simulink model "CasaDi_NMPC_MHE_UGV_circle2m"  (R2022a)
settings: Solver=VariableStepAuto  StartTime=0.0  StopTime=60*2  RelTol=1e-3
values from neighbouring files (symbols this model uses):
  L = 0.14    [MHE_RK_CasaDi.m]    (also in NonLinear_MPC_with_Obstacles_CasaDi.m; SimulationParameters.mat)
  Optitrack_meanerr = [0 0 0]    [SimulationParameters.mat]
  Optitrack_Ts = 0.00833333333333    [SimulationParameters.mat]
  Optitrack_var = [2e-05 2e-05 0.00174532925199]    [SimulationParameters.mat]
  Ts = 0.1    [MHE_RK_CasaDi.m]    (also in NonLinear_MPC_with_Obstacles_CasaDi.m; SimulationParameters.mat)
settings Model: Creator=mrnel  LastModifiedBy=root

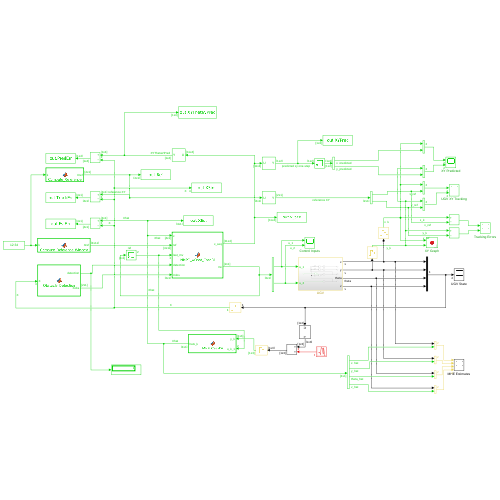
[thumbnail: Simulink's stored preview of the top-level diagram]
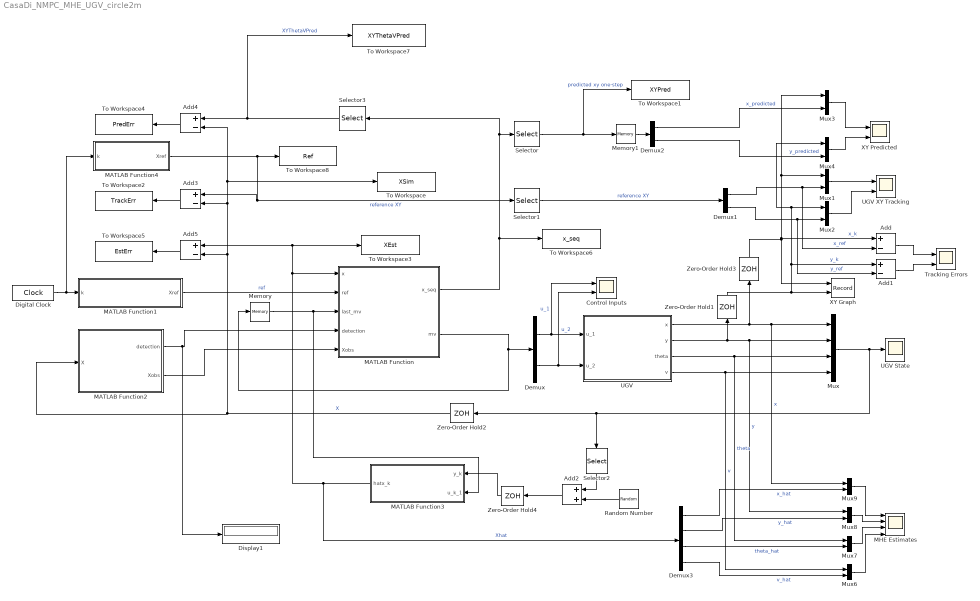
== system CasaDi_NMPC_MHE_UGV_circle2m ==
  Add{,1,3..5} (5 alike) : Sum  Inputs=+-
  Add2 : Sum
  Control Inputs : Scope  NumInputPorts=2
  Demux : Demux  Outputs=2
  Demux1 : Demux  Outputs=2
  Demux2 : Demux  Outputs=2
  Demux3 : Demux
  Digital Clock : DigitalClock  SampleTime=Ts
  Display1 : Display
  MATLAB Function : MATLAB Function  TreatAsAtomicUnit=on  SystemSampleTime=Ts
  MATLAB Function1 : MATLAB Function  TreatAsAtomicUnit=on  SystemSampleTime=Ts
  MATLAB Function2 : MATLAB Function  TreatAsAtomicUnit=on  SystemSampleTime=Ts
  MATLAB Function3 : MATLAB Function  TreatAsAtomicUnit=on  SystemSampleTime=Ts
  MATLAB Function4 : MATLAB Function  TreatAsAtomicUnit=on  SystemSampleTime=Ts
  MHE Estimates : Scope  NumInputPorts=4
  Memory : Memory  InitialCondition=[0;0]  InheritSampleTime=on
  Memory1 : Memory  InitialCondition=[2,0]  InheritSampleTime=on
  Mux : Mux
  Mux{1..4,6..9} (8 alike) : Mux  Inputs=2
  Random Number : RandomNumber  Mean=Optitrack_meanerr  Variance=Optitrack_var.^2  SampleTime=Optitrack_Ts
  Selector : Selector  NumberOfDimensions=2  InputPortWidth=3  IndexOptions=Index vector (dialog),Index vector (dialog)  Indices=2,[1 2]  OutputSizes=1,1
  Selector1 : Selector  NumberOfDimensions=2  InputPortWidth=3  IndexOptions=Index vector (dialog),Index vector (dialog)  Indices=[1 2 ],1  OutputSizes=1,1
  Selector2 : Selector  NumberOfDimensions=2  InputPortWidth=3  IndexOptions=Index vector (dialog),Index vector (dialog)  Indices=1,[1:3]  OutputSizes=1,1
  Selector3 : Selector  NumberOfDimensions=2  InputPortWidth=3  IndexOptions=Index vector (dialog),Select all  Indices=2,[1 2]  OutputSizes=1,1
  To Workspace : ToWorkspace  VariableName=XSim  SaveFormat=Timeseries  SampleTime=Ts
  To Workspace1 : ToWorkspace  VariableName=XYPred  SaveFormat=Timeseries  SampleTime=Ts
  To Workspace2 : ToWorkspace  VariableName=TrackErr  SaveFormat=Timeseries  SampleTime=Ts
  To Workspace3 : ToWorkspace  VariableName=XEst  SaveFormat=Timeseries  SampleTime=Ts
  To Workspace4 : ToWorkspace  VariableName=PredErr  SaveFormat=Timeseries  SampleTime=Ts
  To Workspace5 : ToWorkspace  VariableName=EstErr  SaveFormat=Timeseries  SampleTime=Ts
  To Workspace6 : ToWorkspace  VariableName=x_seq  SaveFormat=Timeseries  SampleTime=-1
  To Workspace7 : ToWorkspace  VariableName=XYThetaVPred  SaveFormat=Timeseries  SampleTime=Ts
  To Workspace8 : ToWorkspace  VariableName=Ref  SaveFormat=Timeseries  SampleTime=Ts
  Tracking Errors : Scope  NumInputPorts=2
  UGV : Subsystem
  UGV State : Scope
  UGV XY Tracking : Scope  NumInputPorts=2
  XY Graph : Record  FileSettingsInternal="{\"entries\":[{\"content\":{\"excelSettings\":{\"content\":{},\"type\":\"Streamout.ExcelSettings\"}},\"type\":\"Streamout.FileSettingStorage\",\"uuid\":\"\"}],\"packageUris\":[\"http:\\/\\/schema.mathworks.com\\/mf0\\/streamout_blocks\\/R2020a\"],\"version\":\"1.0\"}"  Layout=[1 1]  SignalsInternal="{\"entries\":[{\"content\":{\"signals\":[{\"content\":{\"blockPath\":[],\"channel\":[],\"dimensions\":[1,1],\"domain\":\"\",\"lineColor\":\"#a2142f\",\"plots\":[],\"port\":1,\"sid\":[\"\"],\"signalID\":288,\"signalName\":\"x_k\"},\"type\":\"RecordBlkView.Signal\",\"uuid\":\"\"},{\"content\":{\"blockPath\":[],\"channel\":[],\"dimensions\":[1,1],\"domain\":\"\",\"lineColor\":\"#139fff\",\"plots\":[],\"port\":2,\"sid\":[\"\"],\"signalID\":292,\"signalName\":\"y_k\"},\"type\":\"RecordBlkView.Signal\",\"uuid\":\"\"}]},\"type\":\"RecordBlkView.InputSignals\",\"uuid\":\"\"}],\"packageUris\":[\"http:\\/\\/schema.mathworks.com\\/mf0\\/streamout_blocks\\/R2020a\"],\"version\":\"1.0\"}"  VisualizationBindings="{\"xyplotplugin\":{\"info\":[{\"series\":[],\"subplotID\":1}]}}"  CompatibilityTag=XY
  XY Predicted : Scope  NumInputPorts=2
  Zero-Order Hold1 : ZeroOrderHold  SampleTime=Ts
  Zero-Order Hold2 : ZeroOrderHold  SampleTime=Ts
  Zero-Order Hold3 : ZeroOrderHold  SampleTime=Ts
  Zero-Order Hold4 : ZeroOrderHold  SampleTime=0.1
  wires:
  Demux/1 -> UGV/1(u_1), Control Inputs/1  "u_1"
  Demux/2 -> UGV/2("u_2 "), Control Inputs/2  "u_2"
  MATLAB Function/2(mv) -> Demux/1, Memory/1
  Mux/1 -> UGV State/1, Zero-Order Hold2/1, Selector2/1
  Memory/1 -> MATLAB Function3/2(u_k_1), MATLAB Function/3(last_mv)
  UGV/1(x) -> Mux/1, Mux9/1, Zero-Order Hold3/1  "x"
  UGV/2(y) -> Mux/2, Mux8/1, Zero-Order Hold1/1  "y"
  UGV/3(theta) -> Mux/3, Mux7/1  "theta"
  UGV/4(v) -> Mux/4, Mux6/1  "v"
  MATLAB Function/1(x_seq) -> To Workspace6/1, Selector3/1, Selector/1
  Selector/1 -> Memory1/1, To Workspace1/1  "predicted xy one-step"
  Digital Clock/1 -> MATLAB Function4/1(k), MATLAB Function1/1(k)
  Selector1/1 -> Demux1/1  "reference XY"
  Demux2/1 -> Mux3/2  "x_predicted"
  Demux2/2 -> Mux4/2  "y_predicted"
  Mux4/1 -> XY Predicted/2
  Mux3/1 -> XY Predicted/1
  Mux1/1 -> UGV XY Tracking/1
  Mux2/1 -> UGV XY Tracking/2
  Demux1/1 -> Add/2, Mux1/2  "x_ref"
  Demux1/2 -> Mux2/2, Add1/2  "y_ref"
  Zero-Order Hold1/1 -> XY Graph/2, Add1/1, Mux4/1, Mux2/1  "y_k"
  Zero-Order Hold3/1 -> XY Graph/1, Mux3/1, Mux1/1, Add/1  "x_k"
  Add/1 -> Tracking Errors/1
  Add1/1 -> Tracking Errors/2
  MATLAB Function3/1(hatx_k) -> Demux3/1, To Workspace3/1, Add5/1, MATLAB Function/1(x)  "Xhat"
  Add2/1 -> Zero-Order Hold4/1
  Random Number/1 -> Add2/2
  Zero-Order Hold4/1 -> MATLAB Function3/1(y_k)
  Selector2/1 -> Add2/1
  Demux3/1 -> Mux9/2  "x_hat"
  Demux3/2 -> Mux8/2  "y_hat"
  Demux3/3 -> Mux7/2  "theta_hat"
  Demux3/4 -> Mux6/2  "v_hat"
  Mux9/1 -> MHE Estimates/1
  Mux8/1 -> MHE Estimates/2
  Mux7/1 -> MHE Estimates/3
  Mux6/1 -> MHE Estimates/4
  Memory1/1 -> Demux2/1
  Add4/1 -> To Workspace4/1
  Add5/1 -> To Workspace5/1
  Zero-Order Hold2/1 -> Add5/2, Add3/2, To Workspace/1, Add4/2, MATLAB Function2/1(X)  "X"
  Selector3/1 -> To Workspace7/1, Add4/1  "XYThetaVPred"
  MATLAB Function2/1(detection) -> Display1/1, MATLAB Function/4(detection)
  MATLAB Function2/2(Xobs) -> MATLAB Function/5(Xobs)
  MATLAB Function1/1(Xref) -> MATLAB Function/2(ref)  "ref"
  Add3/1 -> To Workspace2/1
  MATLAB Function4/1(Xref) -> To Workspace8/1, Add3/1, Selector1/1  "reference XY"

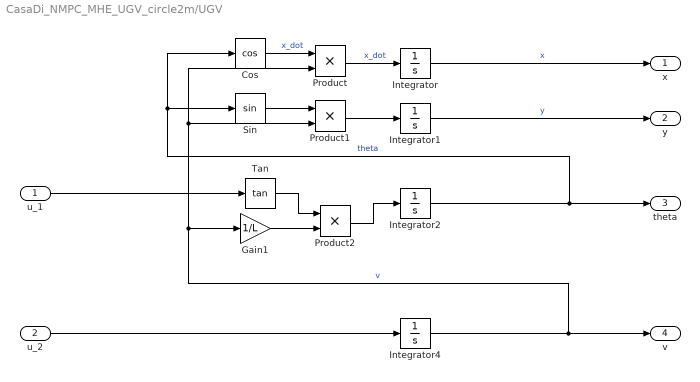
== system CasaDi_NMPC_MHE_UGV_circle2m/UGV ==
  u_1 : Inport
  "u_2 " : Inport  Port=2
  Cos : Trigonometry  Operator=cos
  Gain1 : Gain  Gain=1/L
  Integrator : Integrator  InitialCondition=2
  Integrator1 : Integrator
  Integrator2 : Integrator  InitialCondition=pi/2
  Integrator4 : Integrator  LimitOutput=on  UpperSaturationLimit=1  LowerSaturationLimit=-1
  Product : Product
  Product1 : Product
  Product2 : Product
  Sin : Trigonometry
  Tan : Trigonometry  Operator=tan
  x : Outport
  y : Outport  Port=2
  theta : Outport  Port=3
  v : Outport  Port=4
  wires:
  Product2/1 -> Integrator2/1
  Product1/1 -> Integrator1/1
  Cos/1 -> Product/1  "x_dot"
  Sin/1 -> Product1/1
  Tan/1 -> Product2/1
  Product/1 -> Integrator/1  "x_dot"
  Integrator4/1 -> Product1/2, Product/2, Gain1/1, v/1  "v"
  u_1/1 -> Tan/1
  Integrator1/1 -> y/1  "y"
  "u_2 "/1 -> Integrator4/1
  Integrator/1 -> x/1  "x"
  Integrator2/1 -> Cos/1, Sin/1, theta/1  "theta"
  Gain1/1 -> Product2/2

== matlab function CasaDi_NMPC_MHE_UGV_circle2m/MATLAB Function1 ==
  settings: updateMethod=DISCRETE  sampleTime=Ts
  data: Xref output; k input
function Xref = Compute_Reference_Window(k)
%COMPUTE_REFERENCE_WINDOW This function computes the reference over the prediction
%window, i.e., for instants k, k+1, ..., k+Hp

% Prediction horizon
Hp = 10;

% Time instants over the prediction horizon
time_horizon = k + 0.1 * (0:Hp);

% Intialization of the memory with zeros
Xref = zeros(4,Hp+1);

% Circular trajectory reference for pose and forward velocity. 
w = 2*pi/(60);
Xref = [2*cos(time_horizon*w);
        2*sin(time_horizon*w);
        w*time_horizon+(pi/2);
        2*w*ones(1,Hp+1)];

== matlab function CasaDi_NMPC_MHE_UGV_circle2m/MATLAB Function ==
  data: x input; ref input; last_mv input; x_seq output; mv output; detection input; Xobs input
function [x_seq, mv] = NMPC_wObst_CasaDi(x, ref, last_mv, ...
    detection, Xobs)
%NMPC_WOBST_CASADI This function calls the NMPC function. In particular the
% NMPC formulation includes constraints for obstacle avoidance and the IPOPT
% solver is used to solve the nonlinear optimization problem

% In order to call the 'NonLinear_MPC_with_Obstacles_CasaDi' MATLAB
% Function with the CasaDi library functions calls.
coder.extrinsic("NonLinear_MPC_with_Obstacles_CasaDi");

% Prediction horizon
Hp = 10;

% N. of state variables
n_states = 4;

% N. of control variables
n_controls = 2;

% Initialization of the the memory with zeros of the return values, i.e.,
% * the optimal state sequence over the prediction horizon
x_seq = zeros(Hp+1,n_states);

% * the optimal first control value from the optimal control sequenceover
% the control horizon
mv = zeros(n_controls,1);

% Call of the 'NonLinear_MPC_with_Obstacles_CasaDi' MATLAB function
[x_seq, mv] = NonLinear_MPC_with_Obstacles_CasaDi(x, ref, last_mv, ...
    detection, Xobs);

== matlab function CasaDi_NMPC_MHE_UGV_circle2m/MATLAB Function2 ==
  settings: updateMethod=DISCRETE  sampleTime=Ts
  data: detection output; X input; Xobs output
function [detection, Xobs] = Obstacle_Detection(X)
%OBSTACLE_DETECTION This function implements in some sort the logic of the
% LiDar sensor assumed to be included in the onboard equipment.For
% debugging, a warning is through in case the vehicle enters in the unsafe
% region (i.e., it's too close to the vehicle).

% In order to through a warning if the safety region is not respected
% (i.e., too close to the obstacle)
coder.extrinsic('warning')

% The unknown obstacle is splaced in (x,y) = (-2,0)
Xobs = [-2;0];

% Flag whether an obstacle is detected, 1, or not, 0. By default, no
% obstacle is detected by the LiDar sensor
detection = 0;

% Range of the LiDar sensor.
d_LiDar = 5;%[m]

% Safety distance that the vehicle should keep from the obstacle
d_SAFE = 0.25;%[m]

% If the LiDar onboard detects an obstacle
if norm(X(1:2)-Xobs) < d_LiDar
    % Update the flag 
    detection = 1;
    % If the vehicle enters in the unsafe region ...
    if norm(X(1:2)-Xobs) < d_SAFE
        % ...through a warning...
        warning('too close the obstacle');
        % ...and display the distance from the obstacle (for debugging)
        disp(norm(X(1:2)-Xobs));
    end
end

== matlab function CasaDi_NMPC_MHE_UGV_circle2m/MATLAB Function3 ==
  data: y_k input; hatx_k output; u_k_1 input
function hatx_k = MHE_CasaDi(y_k , u_k_1)
%MHE_CASADI This function calls the MHE function. In particular the IPOPT
% solver is used to solve the nonlinear optimization problem

% In order to call the 'MHE_RK_CasaDi' MATLAB function with the CasaDi 
% library functions calls.
coder.extrinsic("MHE_RK_CasaDi");

% Number of state variables
n_states = 4;

% Number of control variables
n_controls = 2;

% Prediction horizon
N_MHE = 5;

% At each iteration of the MHE, we want to store the batch of previous
% measuments and control inputs and the previous iteration estimate (this
% last is used as initial guess for the IPOPT solver)
persistent y_measurements u_cl X0

% Initialization of persisten values with the initial measurement
if(isempty(y_measurements))
    y0 = [2;0;pi/2];
    y_measurements = repmat(y0,1,N_MHE+1);
end

if(isempty(u_cl))
    % CasaDi wants just one parameter vector, hence added one shadow value 
    % (i.e., below not N_MHE but N_MHE+1) 
    u_cl = zeros(n_controls,N_MHE+1);
end

if(isempty(X0))
    % initialization of the inital guess
    x0 = [2,0,pi/2, 0];
    X0 = repmat(x0,N_MHE+1, 1);
end

% add current measurement
y_measurements = [y_measurements(:,2:end) y_k'];

% add current control input
u_cl = [u_cl(:,2:end-1) u_k_1 u_cl(:,end)];

% call MHE CasaDi function (see the .m file)
X_sol = MHE_RK_CasaDi(y_measurements,u_cl,X0);

% return the estimate of the current state
hatx_k = zeros(n_states,1);
hatx_k = X_sol(N_MHE+1,1:n_states)';

% shift for the next step
X0 = [X_sol(2:(N_MHE+1),1:n_states); X_sol((N_MHE+1),1:n_states)];

end

== matlab function CasaDi_NMPC_MHE_UGV_circle2m/MATLAB Function4 ==
  settings: updateMethod=DISCRETE  sampleTime=Ts
  data: Xref output; k input
function Xref = Compute_Reference(k)
%COMPUTE_REFERNCE This function computes the reference at the current instant k

% Intialization of the memory with zeros
Xref = zeros(4,1);

% Circular trajectory reference for pose and forward velocity. 
w = 2*pi/(60);
Xref = [2*cos(k*w);
        2*sin(k*w);
        w*k+(pi/2);
        2*w];
